simulink model "Example_2"  (R2020b)
settings: Solver=VariableStepAuto  StartTime=0.0  StopTime=0.001  RelTol=1e-3
libraries: fl_lib x13, nesl_utility x5
settings Model: Creator=zaliyazici  LastModifiedBy=zaliyazici

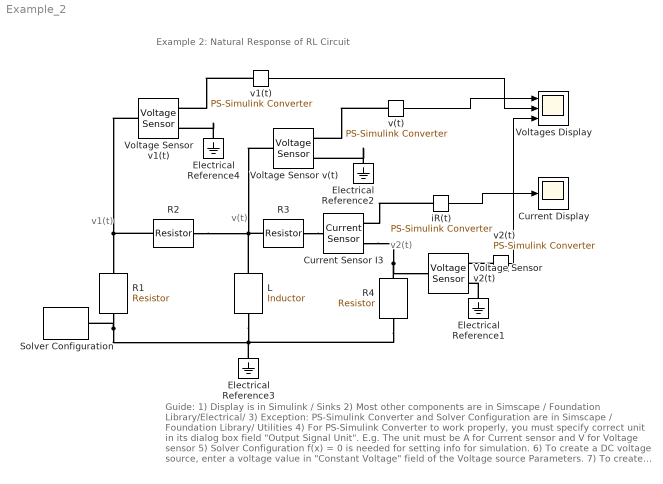
== system Example_2 ==
  note: v2(t)
  note: Guide:
      | 1) Display is in Simulink / Sinks
      | 2) Most other components are in Simscape / Foundation Library/Electrical/
      | 3) Exception: PS-Simulink Converter and Solver Configuration are in Simscape / Foundation Library/ Utilities
      | 4) For PS-Simulink Converter to work properly, you must specify correct unit in its dialog box field "Output Signal Unit".
      | E.g. The unit must be A for Current sensor and V for Voltage sensor
      | 5) Solver Configuration f(x) = 0 is needed for setting info for simulation.
      | 6) To create a DC voltage source, enter a voltage value in "Constant Voltage" field of the Voltage source Parameters.
      | 7) To create "Annotation", double-click a location on project page and select "Create annotation" from the prompt. Then, type any text you want to clarify your circuit. E.g. "Display for Current".
      | 8) To understand how to use a component, right-click on the component and select "Help".
      | Measurement: Node voltages V1(t), v(t), and v1(t), Current through resistor R3 i(t)
  note: Example 2: Natural Response of RL Circuit
  note: v(t)
  note: v1(t)
  Current Display : Scope
  Current Sensor I3 : fl_lib/Electrical/Electrical Sensors/Current Sensor
  Electrical Reference{1..4} (4 alike) : fl_lib/Electrical/Electrical Elements/Electrical Reference
  L : fl_lib/Electrical/Electrical Elements/Inductor  l=100 mH  r=0 Ohm  g=1e-9 1/Ohm  i_specify=off  i_priority=None  i=0 A  i_nominal_specify=off  i_nominal_unit=A  i_nominal_value=1  v_specify=off  v_priority=None  v=0 V  v_nominal_specify=off  v_nominal_unit=V  v_nominal_value=1  i_L_specify=on  i_L_priority=High  i_L=12 mA  i_L_nominal_specify=off  i_L_nominal_unit=A  i_L_nominal_value=1
      settings: AttributesFormatString=|
      | %<l> %<l_unit>
      | %<i_L> %<i_L_unit>
  R1 : fl_lib/Electrical/Electrical Elements/Resistor  R=1 kOhm  i_specify=off  i_priority=None  i=0 A  i_nominal_specify=off  i_nominal_unit=A  i_nominal_value=1  v_specify=off  v_priority=None  v=0 V  v_nominal_specify=off  v_nominal_unit=V  v_nominal_value=1
      settings: AttributesFormatString=%<R> %<R_unit>  LogSimulationData=on
  R2 : fl_lib/Electrical/Electrical Elements/Resistor  R=250 Ohm  i_specify=off  i_priority=None  i=0 A  i_nominal_specify=off  i_nominal_unit=A  i_nominal_value=1  v_specify=off  v_priority=None  v=0 V  v_nominal_specify=off  v_nominal_unit=V  v_nominal_value=1
      settings: AttributesFormatString=%<R> %<R_unit>  LogSimulationData=on
  R3 : fl_lib/Electrical/Electrical Elements/Resistor  R=500 Ohm  i_specify=off  i_priority=None  i=0 A  i_nominal_specify=off  i_nominal_unit=A  i_nominal_value=1  v_specify=off  v_priority=None  v=0 V  v_nominal_specify=off  v_nominal_unit=V  v_nominal_value=1
      settings: AttributesFormatString=%<R> %<R_unit>  LogSimulationData=on
  R4 : fl_lib/Electrical/Electrical Elements/Resistor  R=500 Ohm  i_specify=off  i_priority=None  i=0 A  i_nominal_specify=off  i_nominal_unit=A  i_nominal_value=1  v_specify=off  v_priority=None  v=0 V  v_nominal_specify=off  v_nominal_unit=V  v_nominal_value=1
      settings: AttributesFormatString=%<R> %<R_unit>  LogSimulationData=on
  Solver Configuration : nesl_utility/Solver Configuration  PhysicalDomain=network_engine_domain  SubClassName=solver  LeftPortType=input  RightPortType=generic  Tones=[]  Harmonics=[]  SimulateNoise=off  Profile=off  UseLocalSampling=off  EnableSwitchedLinearOptims=on  FrequencyDomain=off  UseCCode=off  RelTol=0.001  AbsTol=1e-06  MinStep=1e-09  ToWorkspace=off  RevertToSquareIcSolve=off  NumHomotopyIterations=100  PhasorMode=off  PhasorModeNumHarmonics=1  DoDC=off  ResidualTolerance=1e-09  UseLocalSolver=off  LocalSolverChoice=NE_BACKWARD_EULER_ADVANCER  LocalSolverSampleTime=0.001  DoFixedCost=off  MaxNonlinIter=3  MaxModeIter=2  ComputeImpulses=off  ImpulseIterations=2  LinearAlgebra=auto  EquationFormulation=NE_TIME_EF  DelaysMemoryBudget=1024  AutomaticFiltering=on  FilteringTimeConstant=0.001  PartitionStorageMethod=AS_NEEDED  PartitionMemoryBudget=1024  PartitionMethod=ROBUST
  Voltage Sensor v(t) : fl_lib/Electrical/Electrical Sensors/Voltage Sensor
  Voltage Sensor v1(t) : fl_lib/Electrical/Electrical Sensors/Voltage Sensor
  Voltage Sensor v2(t) : fl_lib/Electrical/Electrical Sensors/Voltage Sensor
  Voltages Display : Scope  NumInputPorts=3
  iR(t) : nesl_utility/PS-Simulink Converter  PhysicalDomain=network_engine_domain  SubClassName=ps_output  LeftPortType=input  RightPortType=output  PseudoPeriodic=off  Frequencies=[]  Unit=A  AffineConversion=off
  v(t) : nesl_utility/PS-Simulink Converter  PhysicalDomain=network_engine_domain  SubClassName=ps_output  LeftPortType=input  RightPortType=output  PseudoPeriodic=off  Frequencies=[]  Unit=V  AffineConversion=off
  v1(t) : nesl_utility/PS-Simulink Converter  PhysicalDomain=network_engine_domain  SubClassName=ps_output  LeftPortType=input  RightPortType=output  PseudoPeriodic=off  Frequencies=[]  Unit=V  AffineConversion=off
  v2(t) : nesl_utility/PS-Simulink Converter  PhysicalDomain=network_engine_domain  SubClassName=ps_output  LeftPortType=input  RightPortType=output  PseudoPeriodic=off  Frequencies=[]  Unit=V  AffineConversion=off
  wires:
  v2(t)/1 -> Voltages Display/3
  v(t)/1 -> Voltages Display/1
  iR(t)/1 -> Current Display/1
  v1(t)/1 -> Voltages Display/2
  connections:
  Electrical Reference1/LConn1 -- Voltage Sensor v2(t)/RConn2
  v2(t)/LConn1 -- Voltage Sensor v2(t)/RConn1
  v(t)/LConn1 -- Voltage Sensor v(t)/RConn1
  L/RConn1 -- R3/LConn1 -- R2/LConn1 -- Voltage Sensor v(t)/LConn1
  R4/LConn1 -- Current Sensor I3/RConn2 -- Voltage Sensor v2(t)/LConn1
  Electrical Reference2/LConn1 -- Voltage Sensor v(t)/RConn2
  R1/RConn1 -- Solver Configuration/RConn1 -- L/LConn1 -- Electrical Reference3/LConn1 -- R4/RConn1
  iR(t)/LConn1 -- Current Sensor I3/RConn1
  R3/RConn1 -- Current Sensor I3/LConn1
  R2/RConn1 -- R1/LConn1 -- Voltage Sensor v1(t)/LConn1
  v1(t)/LConn1 -- Voltage Sensor v1(t)/RConn1
  Electrical Reference4/LConn1 -- Voltage Sensor v1(t)/RConn2
